simulink model "PPC"  (R2022b)
settings: Solver=VariableStepAuto  StartTime=0.0  StopTime=151  FixedStep=0.001  RelTol=1e-3
libraries: Solver_SF x1
settings Model: Creator=mzl123  LastModifiedBy=mzl123

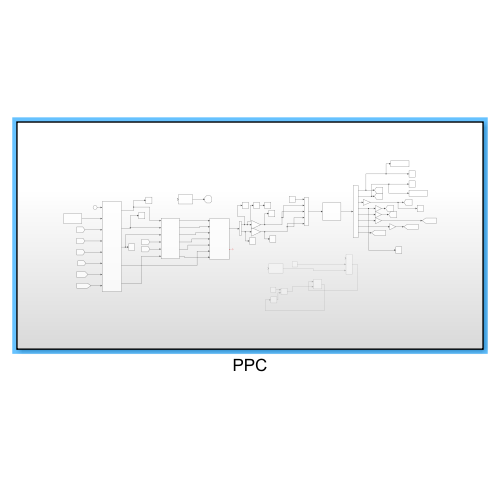
[thumbnail: Simulink's stored preview of the top-level diagram]
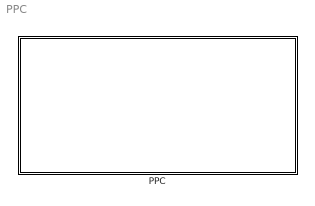
== system PPC ==
  PPC : Subsystem

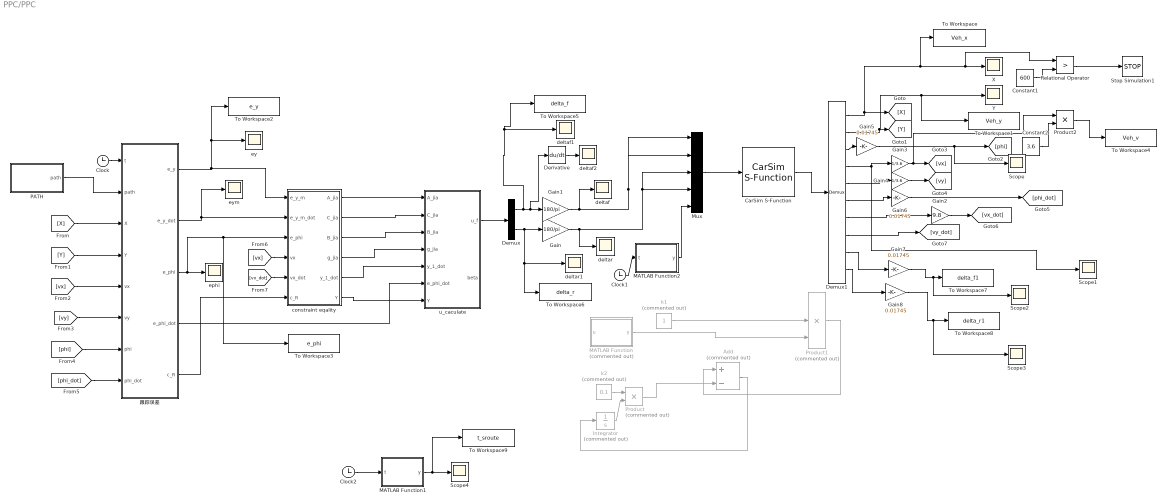
== system PPC/PPC ==
  Add : Sum  Commented=on  Inputs=+-
  CarSim S-Function : Solver_SF/CarSim S-Function  Priority=1  SIMFILE=simfile.sim  Run_RTs=off  vs_state_ind=Run  StopMode_ind=Vehicle Model
  Clock : Clock
  Clock1 : Clock
  Clock2 : Clock
  Constant1 : Constant  Value=600
  Constant2 : Constant  Value=3.6
  Demux : Demux  Outputs=2
  Demux1 : Demux  Outputs=10
  Derivative : Derivative
  Gain : Gain  Gain=180/pi
  Gain1 : Gain  Gain=180/pi
  Gain2 : Gain  Gain=9.8
  Gain3 : Gain  Gain=1/3.6
  Gain4 : Gain  Gain=1/3.6
  Gain{5..8} (4 alike) : Gain  Gain=0.01745
  Integrator : Integrator  Commented=on
  MATLAB Function : MATLAB Function  Commented=on  TreatAsAtomicUnit=on
  MATLAB Function1 : MATLAB Function  TreatAsAtomicUnit=on
  MATLAB Function2 : MATLAB Function  TreatAsAtomicUnit=on
  Mux : Mux  Inputs=5
  PATH : MATLAB Function  TreatAsAtomicUnit=on
  Product : Product  Commented=on
  Product1 : Product  Commented=on  Inputs=3
  Product2 : Product
  Relational Operator : RelationalOperator  Operator=>  OutDataTypeStr=boolean  RndMeth=Simplest  InputSameDT=off
  Scope{,1..4} (5 alike) : Scope
  Stop Simulation1 : Stop
  To Workspace : ToWorkspace  VariableName=Veh_x  SaveFormat=Structure  SampleTime=-1
  To Workspace1 : ToWorkspace  VariableName=Veh_y  SaveFormat=Structure  SampleTime=-1
  To Workspace2 : ToWorkspace  VariableName=e_y  SaveFormat=Structure  SampleTime=-1
  To Workspace3 : ToWorkspace  VariableName=e_phi  SaveFormat=Structure  SampleTime=-1
  To Workspace4 : ToWorkspace  VariableName=Veh_v  SaveFormat=Structure  SampleTime=-1
  To Workspace5 : ToWorkspace  VariableName=delta_f  SaveFormat=Structure With Time  SampleTime=-1
  To Workspace6 : ToWorkspace  VariableName=delta_r  SaveFormat=Structure With Time  SampleTime=-1
  To Workspace7 : ToWorkspace  VariableName=delta_f1  SaveFormat=Structure  SampleTime=-1
  To Workspace8 : ToWorkspace  VariableName=delta_r1  SaveFormat=Structure  SampleTime=-1
  To Workspace9 : ToWorkspace  VariableName=t_sroute  SaveFormat=Structure  SampleTime=-1
  X : Scope
  Y : Scope
  "constraint eqality  " : MATLAB Function  TreatAsAtomicUnit=on
  deltaf : Scope
  deltaf1 : Scope
  deltaf2 : Scope
  deltar : Scope
  deltar1 : Scope
  ephi : Scope
  ey : Scope
  eym : Scope
  k1 : Constant  Commented=on
  k2 : Constant  Commented=on  Value=0.1
  u_caculate : MATLAB Function  TreatAsAtomicUnit=on
  跟踪误差 : MATLAB Function  TreatAsAtomicUnit=on
  wires:
  Demux1/1 -> To Workspace/1, Relational Operator/1, X/1, [X]
  Demux1/2 -> Y/1, To Workspace1/1, [Y]
  "constraint eqality  "/5(y_1_dot) -> u_caculate/5(y_1_dot)
  跟踪误差/5(c_R) -> "constraint eqality  "/6(c_R)
  Demux1/8 -> [vy_dot]
  Gain1/1 -> deltaf/1, Mux/2, Mux/1
  k2/1 -> Product/1
  CarSim S-Function/1 -> Demux1/1
  跟踪误差/3(e_phi) -> To Workspace3/1, "constraint eqality  "/3(e_phi), ephi/1
  Derivative/1 -> deltaf2/1
  "constraint eqality  "/3(B_jia) -> u_caculate/3(B_jia)
  "constraint eqality  "/6(Y) -> u_caculate/7(Y)
  Demux1/5 -> Gain4/1
  Gain5/1 -> Scope/1, [phi]
  "constraint eqality  "/4(g_jia) -> u_caculate/4(g_jia)
  [phi_dot] -> 跟踪误差/8(phi_dot)
  Demux1/3 -> Gain5/1
  Demux/1 -> To Workspace5/1, deltaf1/1, Derivative/1, Gain1/1
  Demux/2 -> To Workspace6/1, deltar1/1, Gain/1
  [vx] -> "constraint eqality  "/4(vx)
  Mux/1 -> CarSim S-Function/1
  [vx] -> 跟踪误差/5(vx)
  Add/1 -> Integrator/1
  Gain6/1 -> [phi_dot]
  MATLAB Function/1(y) -> Product1/3
  PATH/1(path) -> 跟踪误差/2(path)
  Product1/1 -> Add/1
  Gain/1 -> deltar/1, Mux/4, Mux/3
  Product/1 -> Add/2
  Demux1/4 -> Gain3/1, Scope1/1
  [X] -> 跟踪误差/3(X)
  [vy] -> 跟踪误差/6(vy)
  [phi] -> 跟踪误差/7(phi)
  Demux1/7 -> Gain2/1
  "constraint eqality  "/2(C_jia) -> u_caculate/2(C_jia)
  [Y] -> 跟踪误差/4(Y)
  Gain2/1 -> [vx_dot]
  u_caculate/1(u_f) -> Demux/1
  Integrator/1 -> Product/2
  Demux1/6 -> Gain6/1
  k1/1 -> Product1/2
  Clock/1 -> 跟踪误差/1(t)
  [vx_dot] -> "constraint eqality  "/5(vx_dot)
  跟踪误差/4(e_phi_dot) -> u_caculate/6(e_phi_dot)
  Gain3/1 -> Product2/1, [vx]
  Gain4/1 -> [vy]
  "constraint eqality  "/1(A_jia) -> u_caculate/1(A_jia)
  跟踪误差/1(e_y) -> To Workspace2/1, ey/1, "constraint eqality  "/1(e_y_m)
  跟踪误差/2(e_y_dot) -> "constraint eqality  "/2(e_y_m_dot), eym/1
  Constant1/1 -> Relational Operator/2
  Relational Operator/1 -> Stop Simulation1/1
  Constant2/1 -> Product2/2
  Product2/1 -> To Workspace4/1
  Clock1/1 -> MATLAB Function2/1(t)
  MATLAB Function2/1(y) -> Mux/5
  Demux1/9 -> Gain7/1
  Demux1/10 -> Gain8/1
  Gain7/1 -> Scope2/1, To Workspace7/1
  Gain8/1 -> Scope3/1, To Workspace8/1
  Clock2/1 -> MATLAB Function1/1(t)
  MATLAB Function1/1(y) -> To Workspace9/1, Scope4/1

== matlab function PPC/MATLAB Function2 ==
  data: y output; t input
function y = fcn(t)
y = 0.5*0.3*sin(0.2*t);

== matlab function PPC/u_caculate ==
  data: A_jia input; C_jia input; u_f output; B_jia input; g_jia input; y_1_dot input; e_phi_dot input; Y input; beta output
function [u_f,beta] = fcn(A_jia,C_jia,B_jia,g_jia,y_1_dot,e_phi_dot,Y)
b_y = 3;
b_phi =3;
kapha = 13;

Q = [1/b_y 0;
     0   1/b_phi];
Y_dot = [y_1_dot;
         e_phi_dot];
P = [1 0;
     0 1];
beta = Q*Y_dot+Y;


% miu = beta*apha_pie'*men;

% gama = 1/

p_1 = -(B_jia^(-1))*Q*(-1)*(Y_dot+Q*(A_jia*Y_dot+C_jia+g_jia));
% disp(B_jia)
% disp(Q^(-1))
p_2 = -kapha*B_jia^(-1)*Q^(-1)*P^(-1)*beta;
% p_1 = [1;2];
% p_2 = [2;1] ;
% disp(p_1)
% disp(p_2)
% p_3 = -(B_jia^(-1))*Q^(-1)*P^(-1)*gama*miu*apha_pie'*men;
u_f = p_1+p_2;
% disp(u_f)

== matlab function PPC/constraint eqality   ==
  data: e_y_m input; e_y_m_dot input; e_phi input; vx input; A_jia output; vx_dot input; C_jia output; B_jia output; g_jia output; y_1_dot output; Y output; c_R input
function [A_jia,C_jia,B_jia,g_jia,y_1_dot,Y]  = fcn(e_y_m,e_y_m_dot,e_phi,vx,vx_dot,c_R)
%% 车辆参数设计
C_f = 55000;
C_r = 55000;
l_f = 1.015;
l_r = 2.91-1.015;
I_z = 1536;
m = 1412;
e_y_h = 0.2;
e_y_l = -0.2;

%% 动力学矩阵设计
a_1 = (-2*(C_f+C_r))/(m*vx);
a_2 = (-2*(l_f*C_f-l_r*C_r))/(m*vx)-vx;
a_3 = (2*C_f/m);
a_4 = (2*C_r/m);
a_6 = (-2*(l_f*C_f-l_r*C_r))/(I_z*vx);
a_7 = (-2*(l_f^2*C_f+l_r^2*C_r))/(I_z*vx);
a_8 = 2*C_f*l_f/I_z;
a_9 = -2*l_r*C_r/I_z;

A = [a_1  a_2+vx;
     a_6   a_7];
C = [0    -vx*a_1+vx_dot;
     0    -vx*a_6];
g = [vx*c_R*a_2;vx*c_R*a_7-vx_dot*c_R];
B = [a_3 a_4;
     a_8 a_9];


%% 映射变换
gama_1 = pi/(e_y_h-e_y_l);
gama_2 = -pi*(e_y_h+e_y_l)/(2*(e_y_h-e_y_l));
gama_3 = tan(pi*(e_y_h+e_y_l)/(2*(e_y_h-e_y_l)));

%y_1为映射变量
y_1 = tan(gama_1*e_y_m+gama_2)+gama_3;
y_1_dot =(1/((cos(gama_1*e_y_m+gama_2))^2))* gama_1*e_y_m_dot;

kethi_1 = e_y_m;
kethi_2 = 1/(gama_1*(1+(y_1-gama_3)^2));
kethi_3 = -2*y_1_dot*(y_1-gama_3)/(gama_1^2*(1+(y_1-gama_3)^2)^2);

varxi_1 = [kethi_1;
           e_phi];
varxi_2  = [kethi_2 0;0 1];
varxi_3  = [kethi_3 ,0;0,0];

A_jia = (varxi_2^(-1))*A*varxi_2-(varxi_2^(-1))*varxi_3;
C_jia = (varxi_2^(-1))*C*varxi_1;
g_jia = (varxi_2^(-1))*g;
B_jia = (varxi_2^(-1))*B;
Y = [y_1;e_phi];

== matlab function PPC/MATLAB Function ==
  data: u input; y output
function y = fcn(u)

y =norm(u);

== matlab function PPC/跟踪误差 ==
  data: e_y output; e_y_dot output; t input; path input; X input; Y input; vx input; vy input; phi input; phi_dot input; e_phi output; e_phi_dot output; c_R output
% function [e_y,e_y_dot,e_phi,e_phi_dot,c_R] = fcn(t,xr,yr,phi_r,kappar,X,Y,vx,vy,phi,phi_dot)
function [e_y,e_y_dot,e_phi,e_phi_dot,c_R] = fcn(t,path,X,Y,vx,vy,phi,phi_dot)
%% 轨迹处理 
refPos_x = path(:,1);
refPos_y = path(:,2);
refPos = [refPos_x, refPos_y];
pos=[X,Y];
% 计算航向角和曲率
diff_x1 = diff(refPos_x) ;%本质上是一个差分的思想，用后面的减去前面的
diff_x= [diff_x1;diff_x1(end)];
diff_y1 = diff(refPos_y) ;
diff_y = [diff_y1;diff_y1(end)];
derivative1 = gradient(refPos_y) ./ abs(diff_x);              % 一阶导数
derivative2 = del2(refPos_y) ./ abs(diff_x);                  % 二阶导数
derivative3=gradient(del2(refPos_y))./ abs(diff_x); % 三阶导数
refHeading = atan2(diff_y , diff_x);                   % 航向角
refK = abs(derivative2) ./ (1+derivative1.^2).^(3/2);  % 计算曲率
drefK=abs(derivative3+derivative3.*derivative1.^2-3*derivative1.*derivative2.^2)./(1+derivative1.^2).^3; % 计算曲率的导数
%% 首先在参考轨迹上搜索离当前车辆位置最近的点
% 找到距离当前位置最近的一个参考轨迹点的序号
sizeOfrefPos = size(refPos,1);
dist=refPos(:,1);
for i = 1:sizeOfrefPos
    dist(i,1) = norm(refPos(i,:) - pos);   
end
[~,idx] = min(dist); 
% 从该点开始向轨迹前方搜索，找到与预瞄距离最相近的一个轨迹点
     % 从该点开始向轨迹前方搜索，找到与预瞄距离最相近的一个轨迹点
% L_steps = 0;           % 参考轨迹上几个相邻点的累计距离
% % Ld = Kv*v + Ld0;       % Ld0是预瞄距离的下限值；
% Ld =0.5;
% while L_steps < Ld && idx < sizeOfrefPos
%     L_steps = L_steps + norm(refPos(idx + 1,:) - refPos(idx,:));
%     idx = idx+1;
% end
% idx_target = idx;
%% 先找到最近点
% n = length(xr);
% d_min = (X-xr(1))^2+(Y-yr(1))^2;
% min = 1;
% for i=1:n
%       d=(X-xr(i))^2+(Y-yr(i))^2;
%       if d<d_min
%           d_min=d;
%           min=i;
%       end
% end
% idx=min;%找到最近点的路点下标
%% 计算与最近点有关的误差
% e_y=(X-refPos_x(idx))*sin(refHeading(idx))-(Y-refPos_y(idx))*cos(refHeading(idx));
e_y = Y-refPos_y(idx);
e_phi=phi-refHeading(idx);
e_phi_dot=phi_dot-vx*refK(idx);
c_R = refK(idx);
e_y_dot=vy+vx*e_phi;
% c_R_dot=drefK(idx);

%% 误差修正
%  T = 10;
% if ( t <= T)
%     osa = 1-((T-t)/T)^(5);
%     osa_dot = 5*((T-t)/T)^(4)*(1/T);
%     osa_d_dot = -20 * ((T-t)/T)^(3)*(1/(T^2));
% else
%     osa = 1;
%     osa_dot = 0;
%     osa_d_dot = 0;
% end
% kpha = (1-osa+osa_dot*t)*(0.15) + t*(1-osa)*0;
% kpha_dot = (osa_d_dot*t)*(0.15) + (1-osa+osa_dot*t)*0 + (1-osa-t*osa_dot)*(0)+(t-t*osa)*0;
% e_y_m = e_y-kpha ;
% e_y_m_dot = e_y_dot - ((osa_d_dot*t*(0.15))+(1-osa+osa_dot*t)*0)+((1-osa_dot*t-osa)*(0)+(t-osa*t)*0);

== matlab function PPC/PATH ==
  data: path output
function path = path_generation()
%% 直线
% shape=2.4;%参数名称，用于参考轨迹生成
% dx1=25;dx2=21.95;%没有任何实际意义，只是参数名称
% dy1=4.05;dy2=5.7;%没有任何实际意义，只是参数名称
% Xs1=27.19;Xs2=56.46;%参数名称
% X_ref=1:0.1:220;%这个点的区间是根据纵向速度（x_dot）来定的，如果速度为10m/s则区间=10*0.1=1
% z1=shape/dx1*(X_ref-Xs1)-shape/2;
% z2=shape/dx2*(X_ref-Xs2)-shape/2;
% Y_ref=dy1/2.*(1+tanh(z1))-dy2/2.*(1+tanh(z2));
% figure(1);
% plot(X_ref, Y_ref,'r--','LineWidth',2);
% hold on;
% % plot(y.signals.values(:,6),y.signals.values(:,5),'g','LineWidth',2);
% hold off;
%% S线
% X_ref=0:0.1:600;
% n=length(X_ref);
% Y_ref=zeros(1,n);
% Y_ref(1,601:1201)=cos(pi/60.*X_ref(1,601:1201))+1;
% Y_ref(1,1202:4201)=2.*cos(pi/60.*(X_ref(1,1202:4201)-120));
% Y_ref(1,4202:4801)=cos(pi/60.*(X_ref(1,4202:4801)))-1;


% %% 双移线2
X_ref=0:0.1:600;
n=length(X_ref);
Y_ref=zeros(1,n);
Y_ref(1,1001:1501)=1.5*sin(pi/50.*(X_ref(1,1001:1501)-125))+1.5;
Y_ref(1,1502:4501)=3;
Y_ref(1,4502:5001)=1.5.*cos(pi/50.*(X_ref(1,4502:5001)-450))+1.5;
% plot(X_ref(:,1),Y_ref(:,1));

%% 五次多项式曲线
% coefficients = [5.56455900370987e-09,-1.88063163248491e-06,0.000185145086660535,-0.00158567641980212,-0.238324631196854,24.9568568706800];
% X_ref=linspace(0, 100, 1000);
% Y_ref=polyval(coefficients, X_ref);
%% 路径处理
% 
% 计算Y_ref的一阶导数dy/dx (切线斜率)
Y_prime = gradient(Y_ref, X_ref);

% 计算Y_ref的二阶导数d^2y/dx^2
Y_double_prime = gradient(Y_prime, X_ref);

% 计算切线角度theta
theta = atan(Y_prime);

% 计算曲率kappa
kappa = Y_double_prime ./ (1 + Y_prime.^2).^(3/2);

% 定义一个很大的数值来代替无穷大的曲率半径
large_number = 1e6;

% 计算曲率半径R
R = zeros(size(kappa));
for i = 1:length(kappa)
    if abs(kappa(i)) > 1/large_number
        R(i) = 1 / kappa(i);
    else
        R(i) = large_number; % 当曲率接近零时，设为很大的数值
    end
end

% 组合路径数据
path = [X_ref', Y_ref', theta', R', kappa'];


end

== matlab function PPC/MATLAB Function1 ==
  data: t input; y output
function y = fcn(t)

y =20* sin(0.2*t)+40;
